simulink model "PID_controller"  (R2020b)
settings: Solver=VariableStepAuto  StartTime=0.0  StopTime=10.0  RelTol=1e-3
PreLoadFcn:
  | clear all;
  | close all;
  | clc;
  | m=1000;
  | b=50;
  | u=500;
settings Model: Creator=omkar  LastModifiedBy=omkar
settings DataIOCC: SaveOutput=off  SaveTime=off

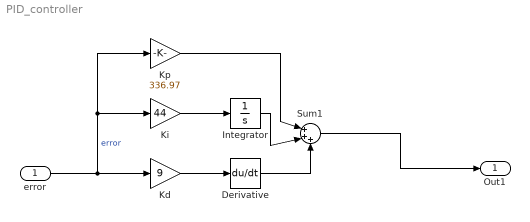
== system PID_controller ==
  error : Inport  OutDataTypeStr=double  PortDimensions=1  SampleTime=0
  Derivative : Derivative
  Integrator : Integrator
  Kd : Gain  Gain=9
  Ki : Gain  Gain=44
  Kp : Gain  Gain=336.97
  Sum1 : Sum  Inputs=|+++
  Out1 : Outport  OutDataTypeStr=double  PortDimensions=1  SampleTime=0
  wires:
  Sum1/1 -> Out1/1
  Kp/1 -> Sum1/1
  Kd/1 -> Derivative/1
  error/1 -> Kd/1, Ki/1, Kp/1  "error"
  Derivative/1 -> Sum1/3
  Integrator/1 -> Sum1/2
  Ki/1 -> Integrator/1
